simulink model "dt_crfb3_non_ideal2"  (R2025b)
settings: Solver=VariableStepAuto  StartTime=0.0  StopTime=30  RelTol=1e-3
model workspace (MAT data in the model file):
  Delay_1 = [0 0 0]
  ENOB_1 = 15.2522734749
  FUNDF_1 = [99.94930421 899.96035216]
  FUNDX_1 = [20.7703735376 -77.1667481387]
  IMODF_1 = [nan nan]
  IMODX_1 = [nan nan]
  NoiseFloor_1 = -107.059481285
  OIP3_1 = nan
  SFDR_1 = 98.8523920816
  SINAD_1 = 93.5786863191
  SNR_1 = 95.0271097041
  THD_1 = -99.0089094369
  delay_1 = [0 0 0]
undefined symbols (not defined in the file): DiscIntNeverNeededParam, Fs
libraries: dspmlti4 x5, msbAdcMeasurements x1, cstblocks x1, dspobslib x1, simulink x1
settings Model: Creator=divya  LastModifiedBy=divya

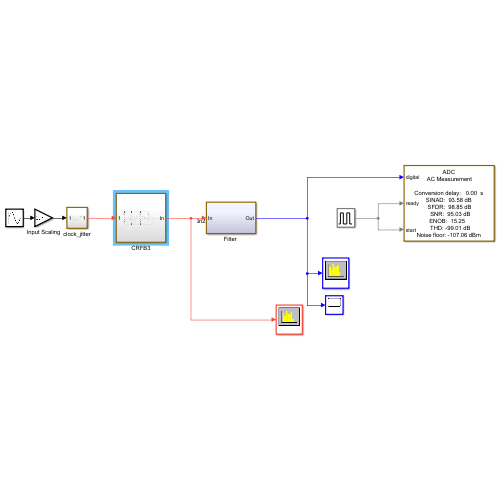
[thumbnail: Simulink's stored preview of the top-level diagram]
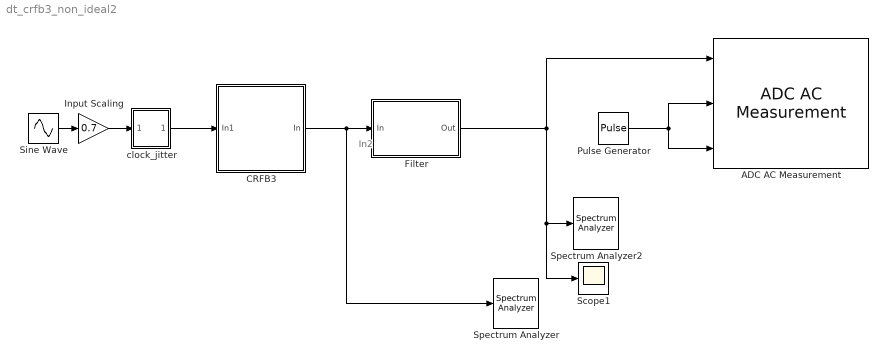
== system dt_crfb3_non_ideal2 ==
  note: In2
  ADC AC Measurement : msbAdcMeasurements/ADC AC Measurement  DistortionMeasurement=Harmonic  InputFrequency=100  Method=Welch (faster, potentially more leakage)  RBW=1.9531  AutoSetRBW=on  NBits=18  Frequency=512e3/256  HoldOffTime=0  OutputToWorkspace=on  VariableName=adc_ac_out  ShowSpectrum=on
      link override ADC AC Measurement/ADC AC Measurement Spectrum Analyzer: YLimits=[-147.2881 39.1044]
  CRFB3 : Subsystem
  "Filter " : Subsystem  Tag=BlockMethodSubSystem
  Input Scaling : Gain  Gain=0.7
  Pulse Generator : DiscretePulseGenerator  PulseType=Time based  Period=1/2e3  PulseWidth=50
  Scope1 : Scope
      settings: ActiveDisplayYMinimum=-0.0095393129139223314  ActiveDisplayYMaximum=0.0095393201553507188
  Sine Wave : Sin  Amplitude=0.7  Frequency=628  SampleTime=0
  Spectrum Analyzer : SpectrumAnalyzer  WindowPosition=[368.000000,182.000000,800.000000,500.000000,]  ScopeFrameLocation=window  WindowInvariantSamplesPerUpdate=on  YLimits=[-98.7682 33.9773]  SelectedToolstripTab=spectrumAnalyzerToolstrip.spectrumTab
  Spectrum Analyzer2 : SpectrumAnalyzer  WindowPosition=[8.000000,20.000000,1520.000000,824.000000,]  ScopeFrameLocation=window  PlotAsTwoSidedSpectrum=off  YLimits=[-58.4541 27.5531]  SelectedToolstripTab=spectrumAnalyzerToolstrip.measurementsTab
  clock_jitter : Subsystem
  wires:
  Sine Wave/1 -> Input Scaling/1
  Input Scaling/1 -> clock_jitter/1(In1)
  Pulse Generator/1 -> ADC AC Measurement/3, ADC AC Measurement/2
  "Filter "/1(Out) -> ADC AC Measurement/1, Scope1/1, Spectrum Analyzer2/1
  clock_jitter/1(Out1) -> CRFB3/1(In1)
  CRFB3/1(In) -> Spectrum Analyzer/1, "Filter "/1(In)

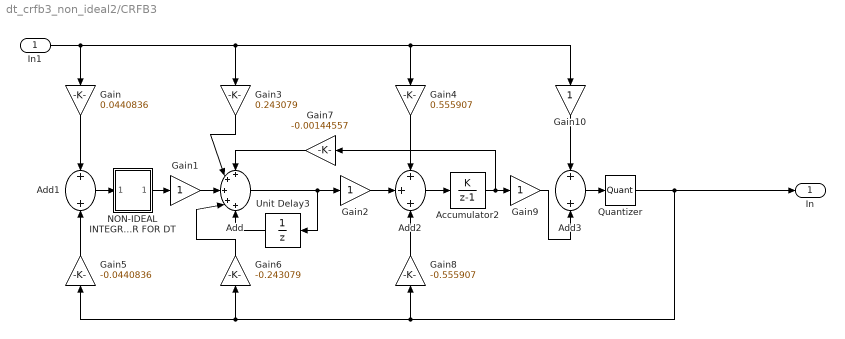
== system dt_crfb3_non_ideal2/CRFB3 ==
  In1 : Inport
  Accumulator2 : DiscreteIntegrator  RequirementInfo={} %GIDa_44cd9c06_0b16_4965_bcb9_a3b882cb6b2b  IntegratorMethod=Accumulation: Forward Euler  SampleTime=-1  ICPrevOutput=DiscIntNeverNeededParam  ICPrevScaledInput=DiscIntNeverNeededParam
  Add : Sum  RequirementInfo={} %GIDa_f157f321_690e_4b54_a3a1_7020e63292c3  Inputs=+++++
  Add1 : Sum  RequirementInfo={} %GIDa_621b426a_3bd7_468e_8275_15c5d793224d
  Add2 : Sum  RequirementInfo={} %GIDa_31058751_ea2a_494a_8028_60e9cd3f5b0a  Inputs=+++
  Add3 : Sum  RequirementInfo={} %GIDa_30c5168d_37b5_410c_ba91_cc520c17976a
  Gain : Gain  RequirementInfo={} %GIDa_90bdcdca_0bd0_492d_a04f_42f19acf9c98  Gain=0.0440836
  Gain1 : Gain  RequirementInfo={} %GIDa_fd1a39f8_4e95_4cec_9b3e_c14353da4ed0
  Gain10 : Gain  RequirementInfo={} %GIDa_bcf9683f_9d2a_47ef_9b9f_3493c12f04e3
  Gain2 : Gain  RequirementInfo={} %GIDa_68d27f5d_a2f8_47fa_a994_19ac67324f44
  Gain3 : Gain  RequirementInfo={} %GIDa_7c82b6a2_4400_4fcb_bb31_cf924035a334  Gain=0.243079
  Gain4 : Gain  RequirementInfo={} %GIDa_9a03bddb_d4e8_4f5c_9644_a14b6e0d4916  Gain=0.555907
  Gain5 : Gain  RequirementInfo={} %GIDa_0e181687_cb7d_467e_a30f_8d65b1326369  Gain=-0.0440836
  Gain6 : Gain  RequirementInfo={} %GIDa_702f2ed7_559a_4a6c_93f7_a3b99cad5188  Gain=-0.243079
  Gain7 : Gain  RequirementInfo={} %GIDa_7c1e3e4a_56b3_4f14_84f4_e15fa2ff8866  Gain=-0.00144557
  Gain8 : Gain  RequirementInfo={} %GIDa_f6fdf6dc_36b9_40d6_a639_f2d4f58e1e13  Gain=-0.555907
  Gain9 : Gain  RequirementInfo={} %GIDa_50be1012_7db1_4aba_ac45_ccbb647d6728
  NON-IDEAL INTEGRATOR FOR DT : Subsystem
  Quantizer : Quantizer  RequirementInfo={} %GIDa_a8f838f2_14c8_491f_8b28_dfa9d167d95c  QuantizationInterval=1
  Unit Delay3 : UnitDelay  SampleTime=-1  HasFrameUpgradeWarning=on
  In : Outport
  wires:
  Gain1/1 -> Add/3
  Add3/1 -> Quantizer/1
  Gain9/1 -> Add3/2
  Add/1 -> Unit Delay3/1, Gain2/1
  Gain4/1 -> Add2/1
  Quantizer/1 -> In/1, Gain8/1, Gain6/1, Gain5/1
  Gain10/1 -> Add3/1
  Gain7/1 -> Add/1
  Add2/1 -> Accumulator2/1
  Accumulator2/1 -> Gain7/1, Gain9/1
  Gain8/1 -> Add2/3
  Gain/1 -> Add1/1
  Unit Delay3/1 -> Add/5
  Gain3/1 -> Add/2
  In1/1 -> Gain/1, Gain3/1, Gain10/1, Gain4/1
  Add1/1 -> NON-IDEAL INTEGRATOR FOR DT/1(In2)
  Gain2/1 -> Add2/2
  Gain5/1 -> Add1/2
  Gain6/1 -> Add/4
  NON-IDEAL INTEGRATOR FOR DT/1(Out1) -> Gain1/1

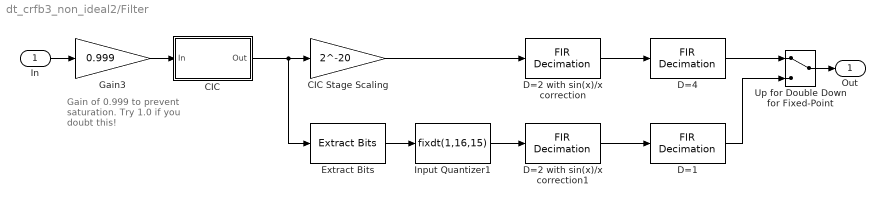
== system dt_crfb3_non_ideal2/Filter  ==
  note: Gain of 0.999
      |  to prevent saturation.
      | Try 1.0 if you doubt this!
  In : Inport
  CIC : Subsystem  Tag=BlockMethodSubSystem
  CIC Stage Scaling : Gain  Gain=2^-20  OutDataTypeStr=double
  D=1 : dspmlti4/FIR Decimation  Tag=BlockMethodSubSystem  FilterSource=Dialog parameters  h=[3.91622882568566e-005 6.87965858042108e-005 -4.54214374064863e-005 -0.000494371495641253 -0.00130180300923401 -0.00208967903904167 -0.00212227242054207 -0.000820466891279789 0.00150204580522739 0.00336930831020411 0.00293785704853453 -0.000377156856911545 -0.00470730589029979 -0.00641725180832836 -0.00285434238807273 0.00468881704747952 0.0106481610663031 0.00886595641260817 -0.00177682957707149 -0.0144760924096176 -0.0180887636371107 -0.00603326390232397 0.0159987454589339 0.0309930177585429 0.0221515825094605 -0.011846123967549 -0.04979943488328 -0.0572170491759349 -0.00847489358036981 0.0923226139783473 0.207458472082029 0.283964644704709 0.283964644704709 0.207458472082029 0.0923226139783473 -0.00847489358036981 -0.0572170491759349 -0.04979943488328 -0.011846123967549 0.0221515825094605 0.0309930177585429 0.0159987454589339 -0.00603326390232397 -0.0180887636371107 -0.0144760924096176 -0.00177682957707149 0.00886595641260817 0.0106481610663031 0.00468881704747952 -0.00285434238807273 -0.00641725180832836 -0.00470730589029979 -0.000377156856911545 0.00293785704853453 0.00336930831020411 0.00150204580522739 -0.000820466891279789 -0.00212227242054207 -0.00208967903904167 -0.00130180300923401 -0.000494371495641253 -4.54214374064863e-005 6.87965858042108e-005 3.91622882568566e-005]  D=4  filtStruct=Direct form  FilterObject=Hm_firdecim  framing=Allow multirate processing  AllowArbitraryInputLength=off  inputOffset=0  outputBufInitCond=0  roundingMode=Floor  overflowMode=off  firstCoeffMode=Binary point scaling  firstCoeffWordLength=16  firstCoeffFracLength=16  firstCoeffDataTypeStr=fixdt(1,16,16)  firstCoeffMin=[]  firstCoeffMax=[]  firstCoeffLastDataTypeStr=fixdt(1,16,16)  outputMin=[]  outputMax=[]
  D=2 with sin(x)/x correction : dspmlti4/FIR Decimation  Tag=BlockMethodSubSystem  FilterSource=Dialog parameters  h=[0.000549322570782159 0.0028188201427819 0.00605408312993028 0.00388745313496409 -0.0121134249050654 -0.0371670852364025 -0.0412525748188521 0.0145135665847005 0.134839839295902 0.264505645586551 0.320972309879795 0.264505645586551 0.134839839295902 0.0145135665847005 -0.0412525748188521 -0.0371670852364025 -0.0121134249050654 0.00388745313496409 0.00605408312993028 0.0028188201427819 0.000549322570782159]  D=2  filtStruct=Direct form  FilterObject=Hm_firdecim  framing=Allow multirate processing  AllowArbitraryInputLength=off  inputOffset=0  outputBufInitCond=0  roundingMode=Floor  overflowMode=off  firstCoeffDataTypeStr=Inherit: Same word length as input  firstCoeffMin=[]  firstCoeffMax=[]  firstCoeffLastDataTypeStr=Inherit: Same word length as input  outputDataTypeStr=Inherit: Same as accumulator  outputMin=[]  outputMax=[]  outputLastDataTypeStr=Inherit: Same as accumulator
  D=2 with sin(x)/x correction1 : dspmlti4/FIR Decimation  Tag=BlockMethodSubSystem  FilterSource=Dialog parameters  h=[0.000549322570782159 0.0028188201427819 0.00605408312993028 0.00388745313496409 -0.0121134249050654 -0.0371670852364025 -0.0412525748188521 0.0145135665847005 0.134839839295902 0.264505645586551 0.320972309879795 0.264505645586551 0.134839839295902 0.0145135665847005 -0.0412525748188521 -0.0371670852364025 -0.0121134249050654 0.00388745313496409 0.00605408312993028 0.0028188201427819 0.000549322570782159]  D=2  filtStruct=Direct form  FilterObject=Hm_firdecim  framing=Allow multirate processing  AllowArbitraryInputLength=off  inputOffset=0  outputBufInitCond=0  roundingMode=Floor  overflowMode=off  firstCoeffMode=Binary point scaling  firstCoeffWordLength=16  firstCoeffFracLength=16  firstCoeffDataTypeStr=fixdt(1,16,16)  firstCoeffMin=[]  firstCoeffMax=[]  firstCoeffLastDataTypeStr=fixdt(1,16,16)  outputMin=[]  outputMax=[]
  D=4 : dspmlti4/FIR Decimation  Tag=BlockMethodSubSystem  FilterSource=Dialog parameters  h=[3.91622882568566e-005 6.87965858042108e-005 -4.54214374064863e-005 -0.000494371495641253 -0.00130180300923401 -0.00208967903904167 -0.00212227242054207 -0.000820466891279789 0.00150204580522739 0.00336930831020411 0.00293785704853453 -0.000377156856911545 -0.00470730589029979 -0.00641725180832836 -0.00285434238807273 0.00468881704747952 0.0106481610663031 0.00886595641260817 -0.00177682957707149 -0.0144760924096176 -0.0180887636371107 -0.00603326390232397 0.0159987454589339 0.0309930177585429 0.0221515825094605 -0.011846123967549 -0.04979943488328 -0.0572170491759349 -0.00847489358036981 0.0923226139783473 0.207458472082029 0.283964644704709 0.283964644704709 0.207458472082029 0.0923226139783473 -0.00847489358036981 -0.0572170491759349 -0.04979943488328 -0.011846123967549 0.0221515825094605 0.0309930177585429 0.0159987454589339 -0.00603326390232397 -0.0180887636371107 -0.0144760924096176 -0.00177682957707149 0.00886595641260817 0.0106481610663031 0.00468881704747952 -0.00285434238807273 -0.00641725180832836 -0.00470730589029979 -0.000377156856911545 0.00293785704853453 0.00336930831020411 0.00150204580522739 -0.000820466891279789 -0.00212227242054207 -0.00208967903904167 -0.00130180300923401 -0.000494371495641253 -4.54214374064863e-005 6.87965858042108e-005 3.91622882568566e-005]  D=4  filtStruct=Direct form  FilterObject=Hm_firdecim  framing=Allow multirate processing  AllowArbitraryInputLength=off  inputOffset=0  outputBufInitCond=0  roundingMode=Floor  overflowMode=off  firstCoeffDataTypeStr=Inherit: Same word length as input  firstCoeffMin=[]  firstCoeffMax=[]  firstCoeffLastDataTypeStr=Inherit: Same word length as input  outputDataTypeStr=Inherit: Same as accumulator  outputMin=[]  outputMax=[]  outputLastDataTypeStr=Inherit: Same as accumulator
  Extract Bits : simulink/Logic and Bit Operations/Extract Bits  bitsToExtract=Upper half  numBits=8  bitIdxRange=[0 7]  outScalingMode=Treat bit field as an integer
  Gain3 : Gain  Gain=0.999
  Input Quantizer1 : DataTypeConversion  OutDataTypeStr=fixdt(1,16,15)  ConvertRealWorld=Stored Integer (SI)  RndMeth=Round
  Up for Double Down for Fixed-Point : ManualSwitch
  Out : Outport  VectorParamsAs1DForOutWhenUnconnected=off
  wires:
  In/1 -> Gain3/1
  CIC/1(Out) -> CIC Stage Scaling/1, Extract Bits/1
  CIC Stage Scaling/1 -> D=2 with sin(x)/x correction/1
  Gain3/1 -> CIC/1(In)
  Input Quantizer1/1 -> D=2 with sin(x)/x correction1/1
  Extract Bits/1 -> Input Quantizer1/1
  D=2 with sin(x)/x correction1/1 -> D=1/1
  D=4/1 -> Up for Double Down for Fixed-Point/1
  D=1/1 -> Up for Double Down for Fixed-Point/2
  Up for Double Down for Fixed-Point/1 -> Out/1
  D=2 with sin(x)/x correction/1 -> D=4/1

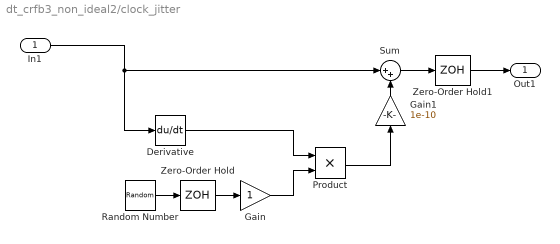
== system dt_crfb3_non_ideal2/clock_jitter ==
  In1 : Inport
  Derivative : Derivative
  Gain : Gain
  Gain1 : Gain  Gain=1e-10
  Product : Product
  Random Number : RandomNumber  SampleTime=0.1
  Sum : Sum  Inputs=|++
  Zero-Order Hold : ZeroOrderHold  SampleTime=-1
  Zero-Order Hold1 : ZeroOrderHold  SampleTime=1/512e3
  Out1 : Outport
  wires:
  In1/1 -> Derivative/1, Sum/1
  Derivative/1 -> Product/1
  Zero-Order Hold1/1 -> Out1/1
  Sum/1 -> Zero-Order Hold1/1
  Random Number/1 -> Zero-Order Hold/1
  Zero-Order Hold/1 -> Gain/1
  Gain/1 -> Product/2
  Gain1/1 -> Sum/2
  Product/1 -> Gain1/1

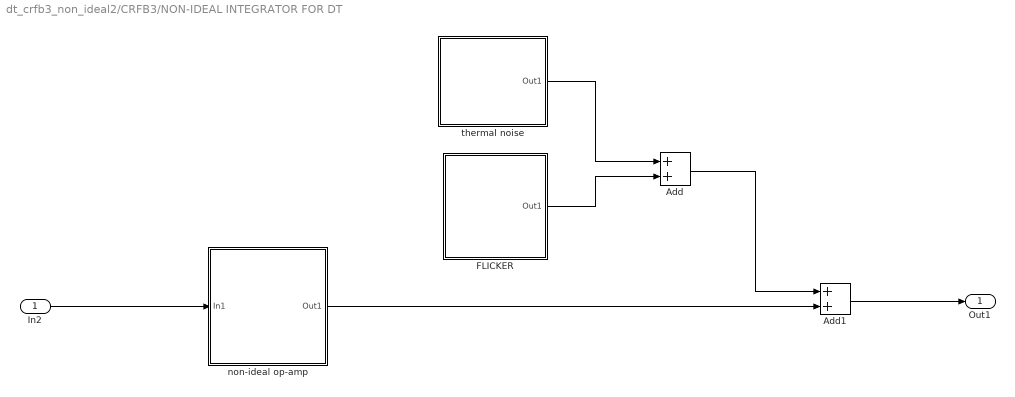
== system dt_crfb3_non_ideal2/CRFB3/NON-IDEAL INTEGRATOR FOR DT ==
  In2 : Inport
  Add : Sum
  Add1 : Sum
  FLICKER : Subsystem
  "non-ideal op-amp " : Subsystem
  thermal noise : Subsystem
  Out1 : Outport
  wires:
  In2/1 -> "non-ideal op-amp "/1(In1)
  Add/1 -> Add1/1
  Add1/1 -> Out1/1
  "non-ideal op-amp "/1(Out1) -> Add1/2
  thermal noise/1(Out1) -> Add/1
  FLICKER/1(Out1) -> Add/2

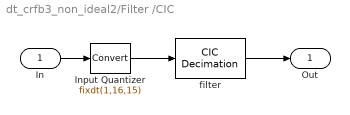
== system dt_crfb3_non_ideal2/Filter /CIC ==
  In : Inport
  Input Quantizer : DataTypeConversion  OutDataTypeStr=fixdt(1,16,15)  RndMeth=Round
  filter : dspmlti4/CIC Decimation  filtFrom=Dialog parameters  filtobj=Hm_decim  ftype=Decimator  R=32  M=1  N=4  filterInternals=Full precision  BPS=[32 32 32 32 32 32 32 32]  FLPS=[15 15 15 15 15 15 15 15]  outputWordLength=32  outputFracLength=15  launchFVT=off  framing=Maintain input frame rate  RateOptions=Allow multirate processing
  Out : Outport  VectorParamsAs1DForOutWhenUnconnected=off
  wires:
  In/1 -> Input Quantizer/1
  Input Quantizer/1 -> filter/1
  filter/1 -> Out/1

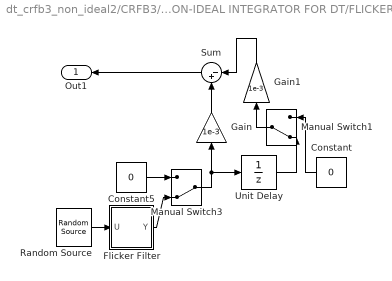
== system dt_crfb3_non_ideal2/CRFB3/NON-IDEAL INTEGRATOR FOR DT/FLICKER ==
  Constant : Constant  Value=0
  Constant5 : Constant  Value=0  SampleTime=1/Fs
  Flicker Filter : Subsystem
  Gain : Gain  Gain=1e-3
  Gain1 : Gain  Gain=1e-3
  Manual Switch1 : ManualSwitch  CurrentSetting=0
  Manual Switch3 : ManualSwitch  CurrentSetting=0
  Random Source : dspobslib/Random Source  SrcType=Gaussian  NormMethod=Ziggurat  CltLength=12  MinVal=0  MaxVal=1  MeanVal=0  VarVal=1  RepMode=Not repeatable  rawSeed=1  IsInherit=off  SampMode=Discrete  SampTime=1/Fs  SampFrame=1  DataType=Double  OutComplex=Real  OutputFrames=off
  Sum : Sum  Inputs=|-+
  Unit Delay : UnitDelay  SampleTime=1/Fs  HasFrameUpgradeWarning=on
  Out1 : Outport
  wires:
  Manual Switch3/1 -> Gain/1, Unit Delay/1
  Random Source/1 -> Flicker Filter/1(U)
  Unit Delay/1 -> Manual Switch1/2
  Constant5/1 -> Manual Switch3/1
  Constant/1 -> Manual Switch1/1
  Gain/1 -> Sum/2
  Flicker Filter/1(Y) -> Manual Switch3/2
  Sum/1 -> Out1/1
  Manual Switch1/1 -> Gain1/1
  Gain1/1 -> Sum/1

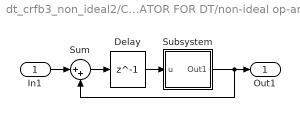
== system dt_crfb3_non_ideal2/CRFB3/NON-IDEAL INTEGRATOR FOR DT/non-ideal op-amp  ==
  In1 : Inport
  Delay : Delay  DelayLength=1  InputProcessing=Columns as channels (frame based)  SampleTime=1/(2e3*256)
  Subsystem : Subsystem
  Sum : Sum  Inputs=|++
  Out1 : Outport
  wires:
  Subsystem/1(Out1) -> Out1/1, Sum/2
  In1/1 -> Sum/1
  Sum/1 -> Delay/1
  Delay/1 -> Subsystem/1(u)

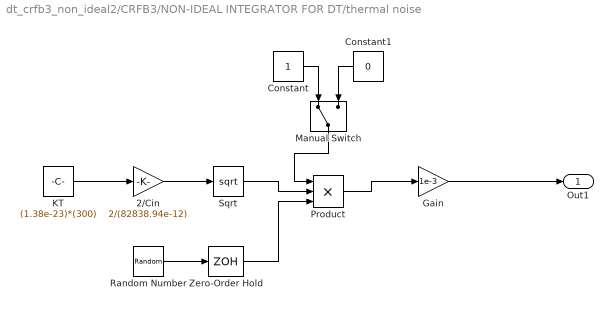
== system dt_crfb3_non_ideal2/CRFB3/NON-IDEAL INTEGRATOR FOR DT/thermal noise ==
  2/Cin : Gain  Gain=2/(82838.94e-12)
  Constant : Constant
  Constant1 : Constant  Value=0
  Gain : Gain  Gain=1e-3
  KT : Constant  Value=(1.38e-23)*(300)
  Manual Switch : ManualSwitch
  Product : Product  Inputs=3
  Random Number : RandomNumber  SampleTime=0.1
  Sqrt : Sqrt
  Zero-Order Hold : ZeroOrderHold  SampleTime=1/(2e3*256)
  Out1 : Outport
  wires:
  Product/1 -> Gain/1
  Random Number/1 -> Zero-Order Hold/1
  KT/1 -> 2/Cin/1
  2/Cin/1 -> Sqrt/1
  Constant1/1 -> Manual Switch/2
  Constant/1 -> Manual Switch/1
  Zero-Order Hold/1 -> Product/3
  Sqrt/1 -> Product/2
  Manual Switch/1 -> Product/1
  Gain/1 -> Out1/1

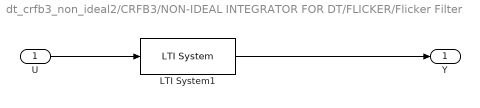
== system dt_crfb3_non_ideal2/CRFB3/NON-IDEAL INTEGRATOR FOR DT/FLICKER/Flicker Filter ==
  U : Inport
  LTI System1 : cstblocks/LTI System  sys=ff_dt  IC=[]  PadeOrder=0
  Y : Outport
  wires:
  LTI System1/1 -> Y/1
  U/1 -> LTI System1/1

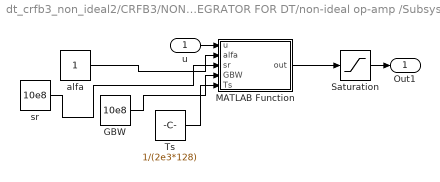
== system dt_crfb3_non_ideal2/CRFB3/NON-IDEAL INTEGRATOR FOR DT/non-ideal op-amp /Subsystem ==
  u : Inport
  GBW : Constant  Value=10e8
  MATLAB Function : MATLAB Function  TreatAsAtomicUnit=on
  Saturation : Saturate  UpperLimit=0.7  LowerLimit=-0.7
  Ts : Constant  Value=1/(2e3*128)
  alfa : Constant
  sr : Constant  Value=10e8
  Out1 : Outport
  wires:
  Ts/1 -> MATLAB Function/5(Ts)
  MATLAB Function/1(out) -> Saturation/1
  alfa/1 -> MATLAB Function/2(alfa)
  GBW/1 -> MATLAB Function/4(GBW)
  sr/1 -> MATLAB Function/3(sr)
  Saturation/1 -> Out1/1
  u/1 -> MATLAB Function/1(u)

== matlab function dt_crfb3_non_ideal2/CRFB3/NON-IDEAL INTEGRATOR FOR DT/non-ideal op-amp /Subsystem/MATLAB Function ==
  data: u input; out output; alfa input; sr input; GBW input; Ts input
function out = slew(u, alfa, sr, GBW, Ts)
% Models the op-amp slew rate for a discrete-time integrator
% u    : input signal amplitude (Vp - Vn)
% alfa : finite gain effect (A0/(1+A0)), ideal op-amp alfa = 1
% sr   : slew rate in V/s
% GBW  : gain-bandwidth of op-amp (Hz)
% Ts   : sample time (s)

tau = 1/(2*pi*GBW);   % time constant
Tmax = Ts/2;           % discrete half-step
slope = alfa * abs(u) / tau;

if slope > sr
    % Op-amp is slewing
    tsl = abs(u)*alfa/sr - tau;   % slewing time
    
    if tsl >= Tmax
        % fully slewing entire half period
        error = abs(u) - sr*Tmax;
    else
        % partial slewing, partial linear region
        texp = Tmax - tsl;
        error = abs(u)*(1-alfa) + (alfa*abs(u) - sr*tsl) * exp(-texp/tau);
    end
    
else
    % Linear region (no slewing)
    texp = Tmax;
    error = abs(u)*(1-alfa) + alfa*abs(u)*exp(-texp/tau);
end

out = u - sign(u)*error;
